simulink model "soal1"  (R2019b)
settings: Solver=VariableStepAuto  StartTime=0.0  StopTime=10  RelTol=1e-3
settings Model: Creator=user  LastModifiedBy=user

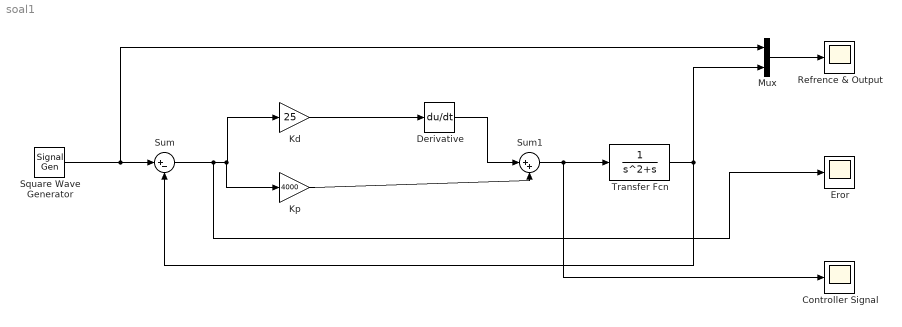
== system soal1 ==
  "Controller Signal " : Scope
  Derivative : Derivative
  "Eror " : Scope
  "Kd " : Gain  Gain=25
  Kp : Gain  Gain=4000
  Mux : Mux  Inputs=2
  Refrence & Output : Scope
  "Square Wave Generator " : SignalGenerator  WaveForm=square  Amplitude=10  Frequency=2.5  Units=rad/sec
  Sum : Sum  Inputs=|+-
  Sum1 : Sum  Inputs=|++
  Transfer Fcn : TransferFcn  Denominator=[1 1 0]
  wires:
  Sum1/1 -> "Controller Signal "/1, Transfer Fcn/1
  Transfer Fcn/1 -> Mux/2, Sum/2
  "Square Wave Generator "/1 -> Mux/1, Sum/1
  Mux/1 -> Refrence & Output/1
  "Kd "/1 -> Derivative/1
  Sum/1 -> "Eror "/1, "Kd "/1, Kp/1
  Kp/1 -> Sum1/2
  Derivative/1 -> Sum1/1
